simulink model "fp_arith_2mul"  (Simulink 7.6)
settings: Solver=ode45  StartTime=0.0  StopTime=1  RelTol=1e-3
settings Model: Creator=jordan  LastModifiedBy=jordan
settings OptimizationCC: BlockReduction=off  ConditionallyExecuteInputs=off

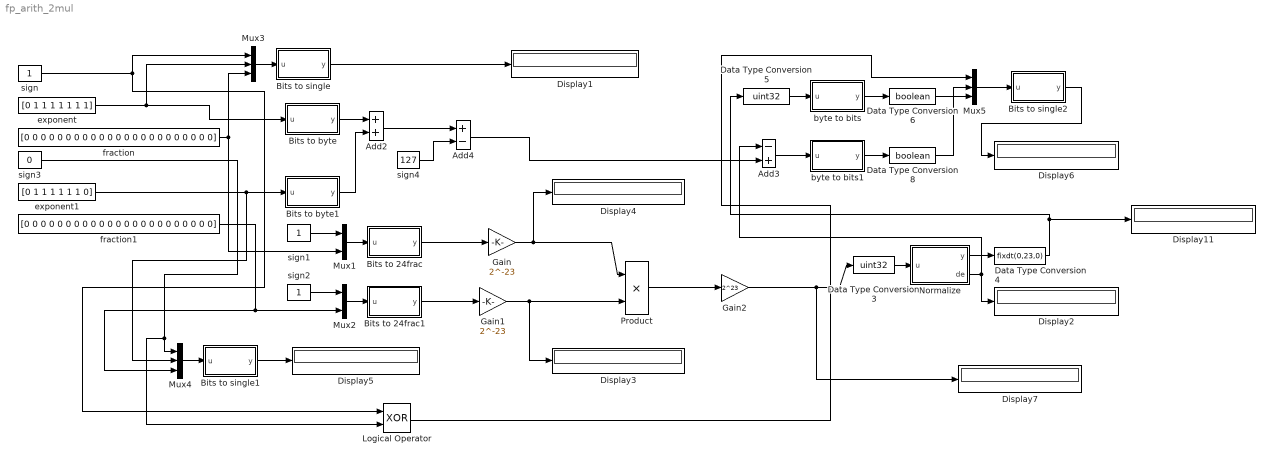
== system fp_arith_2mul ==
  Add2 : Sum  OutDataTypeStr=fixdt(0,9,0)  RndMeth=Nearest
  Add3 : Sum  Inputs=-+  OutDataTypeStr=uint8
  Add4 : Sum  Inputs=+-  OutDataTypeStr=uint8  RndMeth=Nearest
  Bits to 24frac : Stateflow chart  TreatAsAtomicUnit=on
  Bits to 24frac1 : Stateflow chart  TreatAsAtomicUnit=on
  Bits to byte : Stateflow chart  TreatAsAtomicUnit=on
  Bits to byte1 : Stateflow chart  TreatAsAtomicUnit=on
  Bits to single : Stateflow chart  TreatAsAtomicUnit=on
  Bits to single1 : Stateflow chart  TreatAsAtomicUnit=on
  Bits to single2 : Stateflow chart  TreatAsAtomicUnit=on
  Data Type Conversion3 : DataTypeConversion  OutDataTypeStr=uint32
  Data Type Conversion4 : DataTypeConversion  OutDataTypeStr=fixdt(0,23,0)
  Data Type Conversion5 : DataTypeConversion  OutDataTypeStr=uint32
  Data Type Conversion6 : DataTypeConversion  OutDataTypeStr=boolean
  Data Type Conversion8 : DataTypeConversion  OutDataTypeStr=boolean
  Display{1..7,11} (8 alike) : Display
      Display11 settings: Format=hex (Stored Integer)
  Gain : Gain  Gain=2^-23  OutDataTypeStr=fixdt(0,24,23)  RndMeth=Nearest
  Gain1 : Gain  Gain=2^-23  OutDataTypeStr=fixdt(0,24,23)  RndMeth=Nearest
  Gain2 : Gain  Gain=2^23  OutDataTypeStr=fixdt(0,25,0)  RndMeth=Nearest
  Logical Operator : Logic  Operator=XOR  AllPortsSameDT=off  OutDataTypeStr=boolean
  Mux1 : Mux  Inputs=2
  Mux2 : Mux  Inputs=2
  Mux3 : Mux  Inputs=3
  Mux4 : Mux  Inputs=3
  Mux5 : Mux  Inputs=3
  Normalize : Stateflow chart  TreatAsAtomicUnit=on
  Product : Product  OutDataTypeStr=fixdt(0,25,23)  RndMeth=Nearest
  byte to bits : Stateflow chart  TreatAsAtomicUnit=on
  byte to bits1 : Stateflow chart  TreatAsAtomicUnit=on
  exponent : Constant  Value=[0 1 1 1 1 1 1 1]  OutDataTypeStr=boolean
  exponent1 : Constant  Value=[0 1 1 1 1 1 1 0]  OutDataTypeStr=boolean
  fraction : Constant  Value=[0 0 0 0 0 0 0 0 0 0 0 0 0 0 0 0 0 0 0 0 0 0 0]  OutDataTypeStr=boolean
  fraction1 : Constant  Value=[0 0 0 0 0 0 0 0 0 0 0 0 0 0 0 0 0 0 0 0 0 0 0]  OutDataTypeStr=boolean
  sign : Constant  OutDataTypeStr=boolean
  sign1 : Constant  OutDataTypeStr=boolean
  sign2 : Constant  OutDataTypeStr=boolean
  sign3 : Constant  Value=0  OutDataTypeStr=boolean
  sign4 : Constant  Value=127  OutDataTypeStr=fixdt(0,9,0)
  wires:
  exponent/1 -> Bits to byte/1(u), Mux3/2
  fraction/1 -> Mux1/2, Mux3/3
  exponent1/1 -> Bits to byte1/1(u), Mux4/2
  Bits to byte/1(y) -> Add2/1
  Bits to byte1/1(y) -> Add2/2
  Mux1/1 -> Bits to 24frac/1(u)
  sign1/1 -> Mux1/1
  Bits to 24frac/1(y) -> Gain/1
  Mux2/1 -> Bits to 24frac1/1(u)
  sign2/1 -> Mux2/1
  fraction1/1 -> Mux2/2, Mux4/3
  Bits to 24frac1/1(y) -> Gain1/1
  sign/1 -> Mux3/1, Logical Operator/1
  Mux3/1 -> Bits to single/1(u)
  Bits to single/1(y) -> Display1/1
  Mux4/1 -> Bits to single1/1(u)
  sign3/1 -> Mux4/1, Logical Operator/2
  Bits to single1/1(y) -> Display5/1
  Normalize/1(y) -> Data Type Conversion4/1
  Normalize/2(de) -> Display2/1, Add3/1
  Data Type Conversion3/1 -> Normalize/1(u)
  Add3/1 -> byte to bits1/1(u)
  Data Type Conversion4/1 -> Data Type Conversion5/1, Display11/1
  Data Type Conversion5/1 -> byte to bits/1(u)
  byte to bits/1(y) -> Data Type Conversion6/1
  Data Type Conversion6/1 -> Mux5/3
  byte to bits1/1(y) -> Data Type Conversion8/1
  Data Type Conversion8/1 -> Mux5/2
  Mux5/1 -> Bits to single2/1(u)
  Bits to single2/1(y) -> Display6/1
  Logical Operator/1 -> Mux5/1
  Product/1 -> Gain2/1
  Add2/1 -> Add4/1
  sign4/1 -> Add4/2
  Add4/1 -> Add3/2
  Gain/1 -> Product/1, Display4/1
  Gain1/1 -> Product/2, Display3/1
  Gain2/1 -> Display7/1, Data Type Conversion3/1

== matlab function Bits to byte1 ==
  data: u input boolean; y output uint8
function y = fcn(u)
%#eml

u1=uint8(u);
buf=uint8(0);
for ind=1:8
    buf=buf+bitshift(u1(ind),8-ind);
end
y = typecast(buf,'uint8');

== matlab function Bits to 24frac ==
  data: u input boolean; y output uint32
function y = fcn(u)
%#eml

u1=uint32(u);
buf=uint32(0);
for ind=1:24
    buf=buf+bitshift(u1(ind),24-ind);
end
y = buf;

== matlab function Bits to byte ==
  data: u input boolean; y output uint8
function y = fcn(u)
%#eml

u1=uint8(u);
buf=uint8(0);
for ind=1:8
    buf=buf+bitshift(u1(ind),8-ind);
end
y = typecast(buf,'uint8');

== matlab function Bits to 24frac1 ==
  data: u input boolean; y output uint32
function y = fcn(u)
%#eml

u1=uint32(u);
buf=uint32(0);
for ind=1:24
    buf=buf+bitshift(u1(ind),24-ind);
end
y = buf;

== matlab function Bits to single ==
  data: u input boolean; y output single
function y = fcn(u)
%#eml

u1=uint32(u);
buf=uint32(0);
for ind=1:32
    buf=buf+bitshift(u1(ind),32-ind);
end
y = typecast(buf,'single');

== matlab function Bits to single1 ==
  data: u input boolean; y output single
function y = fcn(u)
%#eml

u1=uint32(u);
buf=uint32(0);
for ind=1:32
    buf=buf+bitshift(u1(ind),32-ind);
end
y = typecast(buf,'single');

== matlab function Normalize ==
  data: u input uint32; y output uint32; de output double
function [y,de] = fcn(u)
%#eml

buf=u;
p=int8(-1);
c=bitand(buf,2^24);
for ind=1:25
    if (~c)
        p=p+1;
        buf=bitshift(buf,1);
        c=bitand(buf,2^24);
    end
end
bufy = bitand(bitshift(u,p),2^23-1);
y=bufy;
de=p;

== matlab function byte to bits ==
  data: u input uint32; y output uint8
function y = fcn(u)
%#eml

bufy=uint8(zeros(23,1));
for ind=0:22
    bufy(ind+1)=bitand(bitshift(u,ind),2^22);
end
y=bufy;

== matlab function byte to bits1 ==
  data: u input uint8; y output uint8
function y = fcn(u)
%#eml

bufy=uint8(zeros(8,1));
for ind=0:7
    bufy(ind+1)=bitand(bitshift(u,ind),2^7);
end
y=bufy;

== matlab function Bits to single2 ==
  data: u input boolean; y output single
function y = fcn(u)
%#eml

u1=uint32(u);
buf=uint32(0);
for ind=1:32
    buf=buf+bitshift(u1(ind),32-ind);
end
y = typecast(buf,'single');
